simulink model "untitled2"  (R2021a)
settings: Solver=VariableStepAuto  StartTime=0.0  StopTime=10.0  RelTol=1e-3
libraries: simulink x2
settings Model: Creator=aseghrou  LastModifiedBy=aseghrou

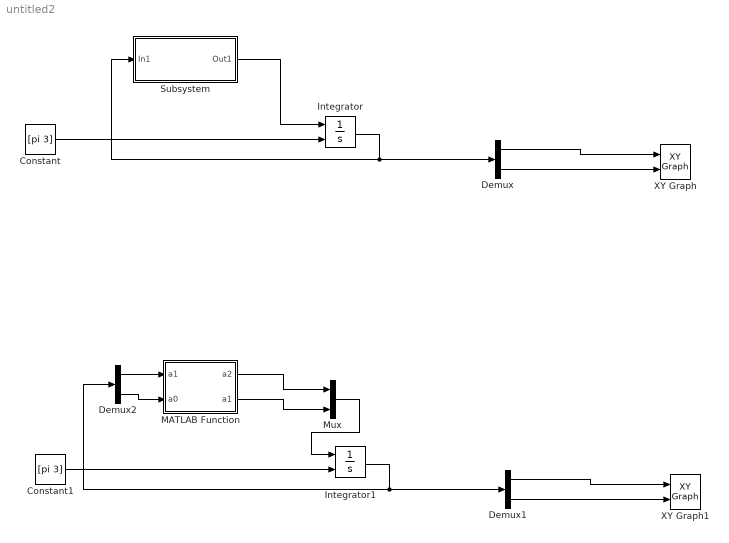
== system untitled2 ==
  Constant : Constant  Value=[pi 3]
  Constant1 : Constant  Value=[pi 3]
  Demux : Demux  Outputs=2
  Demux1 : Demux  Outputs=2
  Demux2 : Demux  Outputs=2
  Integrator : Integrator  InitialConditionSource=external
  Integrator1 : Integrator  InitialConditionSource=external
  MATLAB Function : MATLAB Function  TreatAsAtomicUnit=on
  Mux : Mux  Inputs=2
  Subsystem : Subsystem
  XY Graph : simulink/Sinks/XY Graph  xmin=0  xmax=10  ymin=-2  ymax=10  st=-1
  XY Graph1 : simulink/Sinks/XY Graph  xmin=0  xmax=10  ymin=-2  ymax=10  st=-1
  wires:
  Subsystem/1(Out1) -> Integrator/1
  Integrator/1 -> Subsystem/1(In1), Demux/1
  Constant/1 -> Integrator/2
  MATLAB Function/1(a2) -> Mux/1
  Demux/1 -> XY Graph/1
  Demux/2 -> XY Graph/2
  Demux1/1 -> XY Graph1/1
  Demux1/2 -> XY Graph1/2
  Constant1/1 -> Integrator1/2
  Integrator1/1 -> Demux2/1, Demux1/1
  Demux2/1 -> MATLAB Function/1("a1 ")
  Demux2/2 -> MATLAB Function/2(a0)
  Mux/1 -> Integrator1/1
  MATLAB Function/2(a1) -> Mux/2

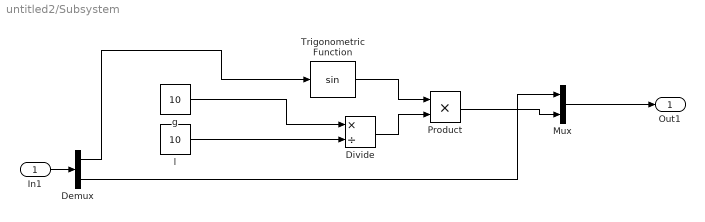
== system untitled2/Subsystem ==
  In1 : Inport
  Demux : Demux  Outputs=2
  Divide : Product  Inputs=*/
  Mux : Mux  Inputs=2
  Product : Product
  Trigonometric Function : Trigonometry
  g : Constant  Value=10
  l : Constant  Value=10
  Out1 : Outport
  wires:
  l/1 -> Divide/2
  g/1 -> Divide/1
  Divide/1 -> Product/2
  Product/1 -> Mux/2
  Trigonometric Function/1 -> Product/1
  Mux/1 -> Out1/1
  In1/1 -> Demux/1
  Demux/1 -> Trigonometric Function/1
  Demux/2 -> Mux/1

== matlab function untitled2/MATLAB Function ==
  data: a1 input; a2 output; a0 input; a1 output
function [a2,a1] = f(a1,a0)

a2 = sin(a0);
